simulink model "singal_three"  (R2023b)
settings: Solver=VariableStepAuto  StartTime=0.0  StopTime=1  RelTol=1e-3
InitFcn:
  | fc=20000;
  | Ts=1/20000;
libraries: spsSeriesRLCBranchLib x17, spsCurrentMeasurementLib x4, spsVoltageMeasurementLib x4, simulink x2, spsUniversalBridgeLib x2, spsDCVoltageSourceLib x1, spsDiodeLib x1, spsMosfetLib x1, spsMutualInductanceLib x1, sps_lib x1
settings Model: SimulationMode=accelerator  Creator=45276  LastModifiedBy=45276

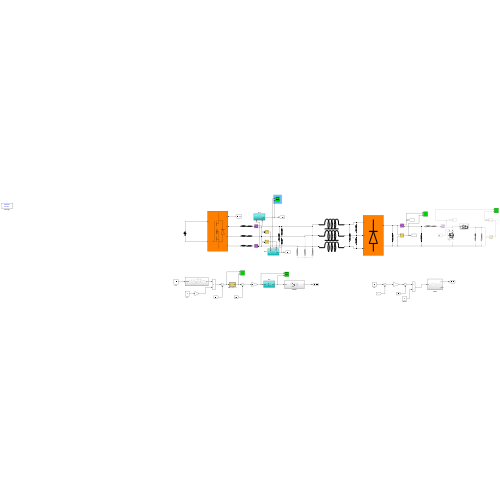
[thumbnail: Simulink's stored preview of the top-level diagram]
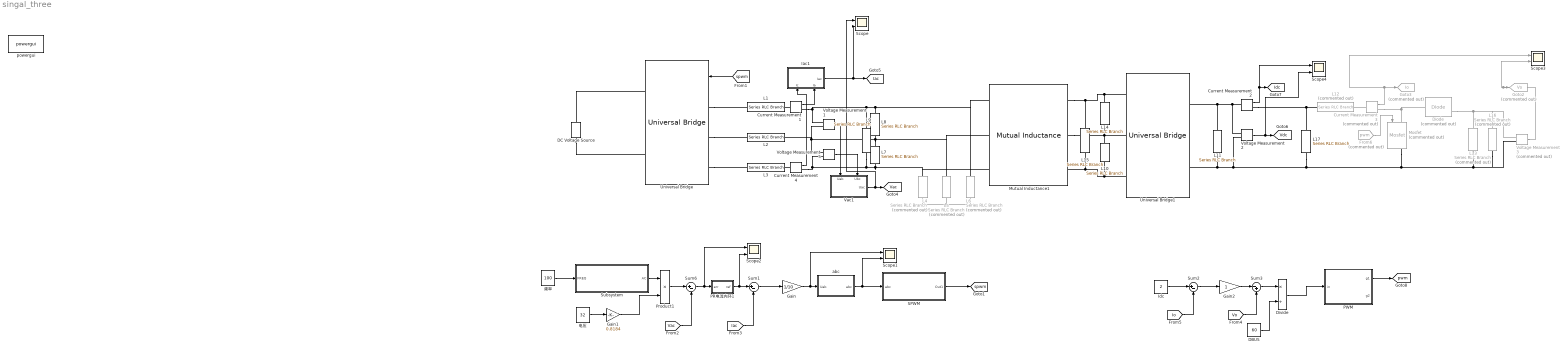
== system singal_three ==
  Current Measurement1 : spsCurrentMeasurementLib/Current Measurement  PhasorSimulation=off  OutputType=Complex  PSBequivalent=0
  Current Measurement2 : spsCurrentMeasurementLib/Current Measurement  PhasorSimulation=off  OutputType=Complex  PSBequivalent=0
  Current Measurement3 : spsCurrentMeasurementLib/Current Measurement  Commented=on  PhasorSimulation=off  OutputType=Complex  PSBequivalent=0
  Current Measurement4 : spsCurrentMeasurementLib/Current Measurement  PhasorSimulation=off  OutputType=Complex  PSBequivalent=0
  DBUS : Constant  Value=60
  DC Voltage Source : spsDCVoltageSourceLib/DC Voltage Source  Amplitude=60  Measurements=None
  Diode : spsDiodeLib/Diode  Commented=on  Ron=0.001  Lon=0  Vf=0.8  IC=0  UseSnubber=0  Rs=500  Cs=250e-9  Measurements=on
  Divide : Product  Inputs=*/
  From6 : From  Commented=on  GotoTag=pwm  TagVisibility=global
  Gain : Gain  Gain=1/10
  Gain1 : Gain  Gain=0.8184
  Gain2 : Gain
  Goto2 : Goto  Commented=on  GotoTag=Vo  TagVisibility=global
  Goto3 : Goto  Commented=on  GotoTag=Io  TagVisibility=global
  Iac1 : Subsystem
      settings: PortSchema="{\"entries\":[{\"content\":{\"sides\":[{\"content\":{\"connectorIds\":[\"In1\",\"In2\"]},\"type\":\"ConnectorPlacement.EquallySpacedRectSide\",\"uuid\":\"58c40194-9a95-4e39-952e-f878bde7484e\"},{\"content\":{\"connectorIds\":[],\"side\":\"RIGHT\"},\"type\":\"ConnectorPlacement.EquallySpacedRectSide\",\"uuid\":\"f51692e8-3ff2-4d72-808d-3667196a4526\"},{\"content\":{\"connectorIds\":[],\"side\":\"TOP\"},\"type\":\"ConnectorPlacement.EquallySpacedRectSide\",\"uuid\":\"0aab136b-5da5-45c4-8998-999ebe8b7f2f\"},{\"content\":{\"connectorIds\":[\"Out1\"],\"side\":\"BOTTOM\"},\"type\":\"ConnectorPlacement.EquallySpacedRectSide\",\"uuid\":\"32f5f4a5-4ebb-496b-828d-b973bd46b44e\"}]},\"type\":\"ConnectorPlacement.EquallySpacedConnector\",\"uuid\":\"3ef81af7-d426-47fb-88e3-e33e58eebb83\"}],\"packageUris\":[\"http://schema.mathworks.com/mf0/Connector/R2020b\"],\"version\":\"1.0\"}"
  Idc : Constant  Value=2
  L1 : spsSeriesRLCBranchLib/Series RLC Branch  LConnTagsString=__new0  RConnTagsString=__new0  BranchType=RL  Resistance=0.001  Inductance=470e-6  SetiL0=off  InitialCurrent=0  Capacitance=3e-6  Setx0=off  InitialVoltage=0  Measurements=None
  L{7..10,14..15} (6 alike) : spsSeriesRLCBranchLib/Series RLC Branch  LConnTagsString=__new0  RConnTagsString=__new0  BranchType=RC  Resistance=0.001  Inductance=2e-3  SetiL0=off  InitialCurrent=0  Capacitance=3e-6  Setx0=off  InitialVoltage=0  Measurements=None
  L11 : spsSeriesRLCBranchLib/Series RLC Branch  LConnTagsString=__new0  RConnTagsString=__new0  BranchType=RC  Resistance=0.001  Inductance=2e-3  SetiL0=off  InitialCurrent=0  Capacitance=3e-3  Setx0=off  InitialVoltage=0  Measurements=None
  L12 : spsSeriesRLCBranchLib/Series RLC Branch  Commented=on  LConnTagsString=__new0  RConnTagsString=__new0  BranchType=RL  Resistance=0.001  Inductance=470e-6  SetiL0=off  InitialCurrent=0  Capacitance=3e-6  Setx0=off  InitialVoltage=0  Measurements=None
  L13 : spsSeriesRLCBranchLib/Series RLC Branch  Commented=on  LConnTagsString=__new0  RConnTagsString=__new0  BranchType=RC  Resistance=0.001  Inductance=2e-3  SetiL0=off  InitialCurrent=0  Capacitance=470e-6  Setx0=off  InitialVoltage=0  Measurements=None
  L16 : spsSeriesRLCBranchLib/Series RLC Branch  Commented=on  LConnTagsString=__new0  RConnTagsString=__new0  BranchType=R  Resistance=20  Inductance=2e-3  SetiL0=off  InitialCurrent=0  Capacitance=470e-6  Setx0=off  InitialVoltage=0  Measurements=None
  L17 : spsSeriesRLCBranchLib/Series RLC Branch  LConnTagsString=__new0  RConnTagsString=__new0  BranchType=R  Resistance=10  Inductance=2e-3  SetiL0=off  InitialCurrent=0  Capacitance=3e-3  Setx0=off  InitialVoltage=0  Measurements=None
  L2 : spsSeriesRLCBranchLib/Series RLC Branch  LConnTagsString=__new0  RConnTagsString=__new0  BranchType=RL  Resistance=0.001  Inductance=470e-6  SetiL0=off  InitialCurrent=0  Capacitance=3e-6  Setx0=off  InitialVoltage=0  Measurements=None
  L3 : spsSeriesRLCBranchLib/Series RLC Branch  LConnTagsString=__new0  RConnTagsString=__new0  BranchType=RL  Resistance=0.001  Inductance=470e-6  SetiL0=off  InitialCurrent=0  Capacitance=3e-6  Setx0=off  InitialVoltage=0  Measurements=None
  L4 : spsSeriesRLCBranchLib/Series RLC Branch  Commented=on  LConnTagsString=__new0  RConnTagsString=__new0  BranchType=R  Resistance=10  Inductance=2e-3  SetiL0=off  InitialCurrent=0  Capacitance=3e-6  Setx0=off  InitialVoltage=0  Measurements=None
  L5 : spsSeriesRLCBranchLib/Series RLC Branch  Commented=on  LConnTagsString=__new0  RConnTagsString=__new0  BranchType=R  Resistance=10  Inductance=2e-3  SetiL0=off  InitialCurrent=0  Capacitance=3e-6  Setx0=off  InitialVoltage=0  Measurements=None
  L6 : spsSeriesRLCBranchLib/Series RLC Branch  Commented=on  LConnTagsString=__new0  RConnTagsString=__new0  BranchType=R  Resistance=10  Inductance=2e-3  SetiL0=off  InitialCurrent=0  Capacitance=3e-6  Setx0=off  InitialVoltage=0  Measurements=None
  Mosfet : spsMosfetLib/Mosfet  Commented=on  Ron=0.1  Lon=0  Rd=0.01  Vfd=0  IC=0  Rs=1e5  Cs=inf  Measurements=on
  Mutual Inductance1 : spsMutualInductanceLib/Mutual Inductance  LConnTagsString=a|b|c  RConnTagsString=A|B|C  TypeOfMutual=Two or three windings with equal mutual terms  NumberOfWindings=3  SelfImpedance1=[0.01 1e-03]  SelfImpedance2=[0.01 1e-03]  ThreeWindings=on  SelfImpedance3=[0.01 1e-03]  MutualImpedance=[0.02 0.9e-03]  InductanceMatrix="[1.0 0.9  0.9 ;  0.9 1.0  0.9;  0.9 0.9 1.0 ] * 1e-3"  ResistanceMatrix="[1.0 0.9  0.9 ;  0.9 1.0  0.9;  0.9 0.9 1.0 ]"  Measurements=None
  PR电流内环1 : Subsystem  TreatAsAtomicUnit=on  mask{Kp=0.1, Kr=40, Wc=10, Upper=40, Lower=-40}
  PWM : Subsystem
  Product1 : Product
  SPWM : Subsystem
  Scope{,1..4} (5 alike) : Scope  NumInputPorts=2
  Subsystem : Subsystem
  Sum1 : Sum  Inputs=|+-
  Sum2 : Sum  Inputs=|+-
  Sum3 : Sum  Inputs=|-+
  Sum6 : Sum  Inputs=|+-
  Universal Bridge : spsUniversalBridgeLib/Universal Bridge  Arms=3  SnubberResistance=1e5  SnubberCapacitance=inf  Device=MOSFET / Diodes  Ron=1e-3  Lon=0  ForwardVoltages="[  0  0  ]"  ForwardVoltage=0  GTOparameters=[ 10e-6 , 20e-6 ]  IGBTparameters=[ 1e-6 , 2e-6 ]  Measurements=None  Measurements_2=None  converterType=Rectifier
  Universal Bridge1 : spsUniversalBridgeLib/Universal Bridge  Arms=3  SnubberResistance=1e5  SnubberCapacitance=inf  Device=Diodes  Ron=1e-3  Lon=0  ForwardVoltages="[  0  0  ]"  ForwardVoltage=0  GTOparameters=[ 10e-6 , 20e-6 ]  IGBTparameters=[ 1e-6 , 2e-6 ]  Measurements=None  Measurements_2=None  converterType=Rectifier
  Vac1 : Subsystem
      settings: PortSchema="{\"entries\":[{\"content\":{\"sides\":[{\"content\":{\"connectorIds\":[\"In1\",\"In2\"]},\"type\":\"ConnectorPlacement.EquallySpacedRectSide\",\"uuid\":\"58c40194-9a95-4e39-952e-f878bde7484e\"},{\"content\":{\"connectorIds\":[],\"side\":\"RIGHT\"},\"type\":\"ConnectorPlacement.EquallySpacedRectSide\",\"uuid\":\"f51692e8-3ff2-4d72-808d-3667196a4526\"},{\"content\":{\"connectorIds\":[],\"side\":\"TOP\"},\"type\":\"ConnectorPlacement.EquallySpacedRectSide\",\"uuid\":\"0aab136b-5da5-45c4-8998-999ebe8b7f2f\"},{\"content\":{\"connectorIds\":[\"Out1\"],\"side\":\"BOTTOM\"},\"type\":\"ConnectorPlacement.EquallySpacedRectSide\",\"uuid\":\"185ce796-68e2-4136-8080-97dc86d2ba54\"}]},\"type\":\"ConnectorPlacement.EquallySpacedConnector\",\"uuid\":\"3ef81af7-d426-47fb-88e3-e33e58eebb83\"}],\"packageUris\":[\"http://schema.mathworks.com/mf0/Connector/R2020b\"],\"version\":\"1.0\"}"
  Voltage Measurement1 : spsVoltageMeasurementLib/Voltage Measurement  PhasorSimulation=off  OutputType=Complex  PSBequivalent=0
  Voltage Measurement2 : spsVoltageMeasurementLib/Voltage Measurement  PhasorSimulation=off  OutputType=Complex  PSBequivalent=0
  Voltage Measurement3 : spsVoltageMeasurementLib/Voltage Measurement  Commented=on  PhasorSimulation=off  OutputType=Complex  PSBequivalent=0
  Voltage Measurement5 : spsVoltageMeasurementLib/Voltage Measurement  PhasorSimulation=off  OutputType=Complex  PSBequivalent=0
  abc : Subsystem
      settings: PortSchema="{\"entries\":[{\"content\":{\"sides\":[{\"content\":{},\"type\":\"ConnectorPlacement.EquallySpacedRectSide\",\"uuid\":\"58c40194-9a95-4e39-952e-f878bde7484e\"},{\"content\":{\"side\":\"RIGHT\"},\"type\":\"ConnectorPlacement.EquallySpacedRectSide\",\"uuid\":\"f51692e8-3ff2-4d72-808d-3667196a4526\"},{\"content\":{\"connectorIds\":[\"In1\"],\"side\":\"TOP\"},\"type\":\"ConnectorPlacement.EquallySpacedRectSide\",\"uuid\":\"0aab136b-5da5-45c4-8998-999ebe8b7f2f\"},{\"content\":{\"connectorIds\":[\"Out1\"],\"side\":\"BOTTOM\"},\"type\":\"ConnectorPlacement.EquallySpacedRectSide\",\"uuid\":\"32f5f4a5-4ebb-496b-828d-b973bd46b44e\"}]},\"type\":\"ConnectorPlacement.EquallySpacedConnector\",\"uuid\":\"3ef81af7-d426-47fb-88e3-e33e58eebb83\"}],\"packageUris\":[\"http://schema.mathworks.com/mf0/Connector/R2020b\"],\"version\":\"1.0\"}"
  powergui : sps_lib/powergui  Priority=1  SimulationMode=Discrete  SampleTime=2e-7  frequency=60  Iterations=50  frequencyindice=0  Pbase=100e6  ErrMax=1e-4  UnitsV=kV  UnitsW=MW  buscounter=0  FunctionMessages=off  echomessages=off  EnableUseOfTLC=off  CurrentSourceSwitches=off  DisableSnubberDevices=off  DisableRonSwitches=off  DisableVfSwitches=off  DisplayEquations=off  AutomaticDiscreteSolvers=off  SolverType=Tustin/Backward Euler (TBE)  Interpol=off  ExternalGateDelay=off  methode=off  Ts=100  x0status=blocks  SPID=on  SwTol=0  HookPort=off  NonlinearTolerance=1e-4  nMaxIteration=100  ContinueOnMaxIteration=off  RestoreLinks=warning  ResistiveCurrentMeasurement=off  Frange=[0:2:500]  Ylog=off  Xlog=on  ShowGrid=off  save=off  variable=ZData  structure=0  ZoomFFT=off  StartTime=0.0  cycles=1  DisplayStyle=1  fundamental=60  FreqAxis=off  MaxFrequency=1000  frequencyindicesteady=1  RmsSteady=1  display=off
  电压 : Constant  Value=32
  频率 : Constant  Value=100
  tag scope: Iac=global, Idc=global, Vac=global, Vdc=global, pwm=global, spwm=global
  wires:
  [spwm] -> Universal Bridge/1
  频率/1 -> Subsystem/1(FREQ)
  Subsystem/1(AC) -> Product1/1
  PR电流内环1/1(ref) -> Scope2/2, Sum1/1
  Sum6/1 -> Scope2/1, PR电流内环1/1(err)
  Product1/1 -> Sum6/1
  电压/1 -> Gain1/1
  Vac1/1(Uac) -> Scope/1, [Vac]
  Voltage Measurement5/1 -> Vac1/2(Ubc)
  Iac1/1(Iac) -> Scope/2, [Iac]
  Voltage Measurement1/1 -> Vac1/1(Uab)
  Current Measurement1/1 -> Iac1/2(Ia)
  Current Measurement4/1 -> Iac1/1(Ic)
  [Vac] -> Sum6/2
  [Iac] -> Sum1/2
  Sum1/1 -> Gain/1
  SPWM/1(Out1) -> [spwm]
  Gain/1 -> Scope1/1, abc/1(Uab)
  abc/1(abc) -> SPWM/1(abc), Scope1/2
  Voltage Measurement3/1 -> Scope3/2, Goto2/1
  Current Measurement3/1 -> Scope3/1, Goto3/1
  Voltage Measurement2/1 -> Scope4/2, [Vdc]
  Current Measurement2/1 -> Scope4/1, [Idc]
  [Io] -> Sum2/2
  Sum2/1 -> Gain2/1
  Divide/1 -> PWM/1(in)
  PWM/1(g1) -> [pwm]
  From6/1 -> Mosfet/1
  Idc/1 -> Sum2/1
  Gain2/1 -> Sum3/1
  Sum3/1 -> Divide/1
  [Vo] -> Sum3/2
  DBUS/1 -> Divide/2
  Gain1/1 -> Product1/2
  connections:
  Universal Bridge/LConn3 -- L3/RConn1
  Universal Bridge/LConn2 -- L2/RConn1
  Universal Bridge/LConn1 -- L1/RConn1
  L7/RConn1 -- Mutual Inductance1/LConn3 -- L4/LConn1 -- L9/RConn1 -- Voltage Measurement5/LConn2 -- Current Measurement4/RConn1
  L8/LConn1 -- L6/LConn1 -- Mutual Inductance1/LConn1 -- L9/LConn1 -- Current Measurement1/RConn1 -- Voltage Measurement1/LConn1
  L7/LConn1 -- Mutual Inductance1/LConn2 -- L5/LConn1 -- L8/RConn1 -- Voltage Measurement1/LConn2 -- L2/LConn1 -- Voltage Measurement5/LConn1
  DC Voltage Source/LConn1 -- Universal Bridge/RConn2
  Current Measurement1/LConn1 -- L1/LConn1
  Current Measurement4/LConn1 -- L3/LConn1
  Voltage Measurement2/LConn1 -- Current Measurement2/LConn1 -- L11/LConn1 -- Universal Bridge1/RConn1
  Current Measurement2/RConn1 -- L17/LConn1 -- L12/RConn1
  Diode/LConn1 -- Current Measurement3/RConn1 -- Mosfet/LConn1
  DC Voltage Source/RConn1 -- Universal Bridge/RConn1
  Current Measurement3/LConn1 -- L12/LConn1
  Mutual Inductance1/RConn1 -- L15/LConn1 -- L14/LConn1 -- Universal Bridge1/LConn1
  Mutual Inductance1/RConn2 -- L14/RConn1 -- L10/LConn1 -- Universal Bridge1/LConn2
  Universal Bridge1/LConn3 -- L10/RConn1 -- L15/RConn1 -- Mutual Inductance1/RConn3
  Diode/RConn1 -- L16/LConn1 -- Voltage Measurement3/LConn1 -- L13/LConn1
  L11/RConn1 -- L17/RConn1 -- L16/RConn1 -- Voltage Measurement3/LConn2 -- L13/RConn1 -- Mosfet/RConn1 -- Voltage Measurement2/LConn2 -- Universal Bridge1/RConn2
  L4/RConn1 -- L5/RConn1 -- L6/RConn1

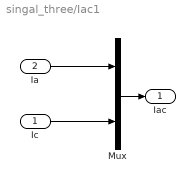
== system singal_three/Iac1 ==
  Ic : Inport
  Ia : Inport  Port=2
  Mux : Mux  Inputs=2
  Iac : Outport
  wires:
  Mux/1 -> Iac/1
  Ic/1 -> Mux/2
  Ia/1 -> Mux/1

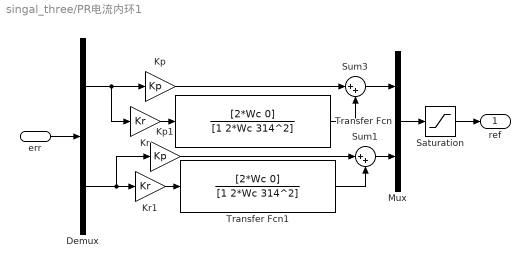
== system singal_three/PR电流内环1 ==
  err : Inport
  Demux : Demux  Outputs=2
  Kp : Gain  Gain=Kp
  Kp1 : Gain  Gain=Kp
  Kr : Gain  Gain=Kr
  Kr1 : Gain  Gain=Kr
  Mux : Mux  Inputs=2
  Saturation : Saturate  UpperLimit=Upper  LowerLimit=Lower
  Sum1 : Sum  Inputs=|++
  Sum3 : Sum  Inputs=|++
  Transfer Fcn : TransferFcn  Numerator=[2*Wc 0]  Denominator=[1 2*Wc 314^2]
  Transfer Fcn1 : TransferFcn  Numerator=[2*Wc 0]  Denominator=[1 2*Wc 314^2]
  ref : Outport
  wires:
  Mux/1 -> Saturation/1
  Sum1/1 -> Mux/2
  Kr1/1 -> Transfer Fcn1/1
  Transfer Fcn1/1 -> Sum1/2
  Kp1/1 -> Sum1/1
  Demux/2 -> Kp1/1, Kr1/1
  Sum3/1 -> Mux/1
  Demux/1 -> Kp/1, Kr/1
  err/1 -> Demux/1
  Kp/1 -> Sum3/1
  Saturation/1 -> ref/1
  Transfer Fcn/1 -> Sum3/2
  Kr/1 -> Transfer Fcn/1

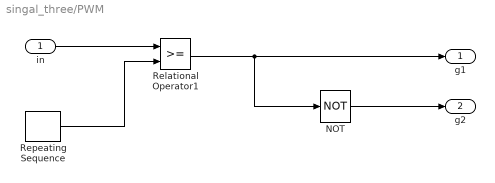
== system singal_three/PWM ==
  in : Inport
  NOT : Logic  Operator=NOT  IconShape=distinctive  AllPortsSameDT=off  OutDataTypeStr=boolean
  Relational Operator1 : RelationalOperator  OutDataTypeStr=boolean  RndMeth=Simplest  InputSameDT=off
  Repeating Sequence : simulink/Sources/Repeating Sequence  rep_seq_t=[0 20000/2 20000]  rep_seq_y=[0 1 0]
  g1 : Outport
  g2 : Outport  Port=2
  wires:
  Relational Operator1/1 -> g1/1, NOT/1
  in/1 -> Relational Operator1/1
  Repeating Sequence/1 -> Relational Operator1/2
  NOT/1 -> g2/1

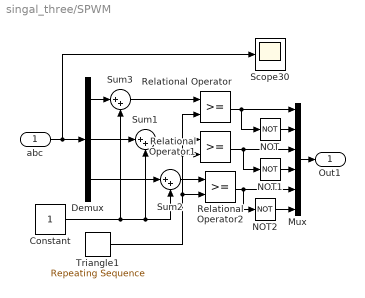
== system singal_three/SPWM ==
  abc : Inport
  Constant : Constant
  Demux : Demux  Outputs=3
  Mux : Mux  Inputs=6
  NOT : Logic  Operator=NOT  IconShape=distinctive  AllPortsSameDT=off  OutDataTypeStr=boolean
  NOT1 : Logic  Operator=NOT  IconShape=distinctive  AllPortsSameDT=off  OutDataTypeStr=boolean
  NOT2 : Logic  Operator=NOT  IconShape=distinctive  AllPortsSameDT=off  OutDataTypeStr=boolean
  Relational Operator : RelationalOperator  OutDataTypeStr=boolean  RndMeth=Simplest  InputSameDT=off
  Relational Operator1 : RelationalOperator  OutDataTypeStr=boolean  RndMeth=Simplest  InputSameDT=off
  Relational Operator2 : RelationalOperator  OutDataTypeStr=boolean  RndMeth=Simplest  InputSameDT=off
  Scope30 : Scope
  Sum1 : Sum  Inputs=|++
  Sum2 : Sum  Inputs=|++
  Sum3 : Sum  Inputs=|++
  Triangle1 : simulink/Sources/Repeating Sequence  rep_seq_t=[0 1/20000/2 1/20000]  rep_seq_y=[0 2 0]
  Out1 : Outport
  wires:
  Mux/1 -> Out1/1
  NOT2/1 -> Mux/6
  NOT1/1 -> Mux/4
  Relational Operator2/1 -> Mux/5, NOT2/1
  Relational Operator1/1 -> Mux/3, NOT1/1
  Relational Operator/1 -> Mux/1, NOT/1
  NOT/1 -> Mux/2
  Triangle1/1 -> Relational Operator/2, Relational Operator1/2, Relational Operator2/2
  abc/1 -> Scope30/1, Demux/1
  Demux/1 -> Sum3/1
  Sum3/1 -> Relational Operator/1
  Demux/2 -> Sum1/1
  Sum1/1 -> Relational Operator1/1
  Demux/3 -> Sum2/1
  Sum2/1 -> Relational Operator2/1
  Constant/1 -> Sum2/2, Sum1/2, Sum3/2

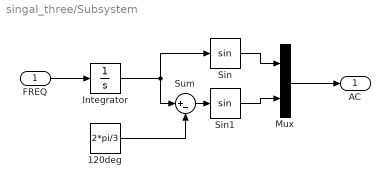
== system singal_three/Subsystem ==
  FREQ : Inport
  120deg : Constant  Value=2*pi/3
  Integrator : Integrator  WrapState=on  WrappedStateUpperValue=2*pi  WrappedStateLowerValue=0
  Mux : Mux  Inputs=2
  Sin : Trigonometry
  Sin1 : Trigonometry
  Sum : Sum  Inputs=|+-
  AC : Outport
  wires:
  FREQ/1 -> Integrator/1
  Sin/1 -> Mux/1
  Mux/1 -> AC/1
  120deg/1 -> Sum/2
  Integrator/1 -> Sin/1, Sum/1
  Sum/1 -> Sin1/1
  Sin1/1 -> Mux/2

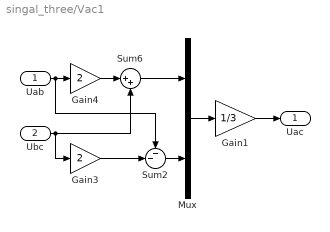
== system singal_three/Vac1 ==
  Uab : Inport
  Ubc : Inport  Port=2
  Gain1 : Gain  Gain=1/3
  Gain3 : Gain  Gain=2
  Gain4 : Gain  Gain=2
  Mux : Mux  Inputs=2
  Sum2 : Sum  Inputs=--|
  Sum6 : Sum  Inputs=|++
  Uac : Outport
  wires:
  Gain1/1 -> Uac/1
  Mux/1 -> Gain1/1
  Gain3/1 -> Sum2/2
  Sum2/1 -> Mux/2
  Ubc/1 -> Gain3/1, Sum6/2
  Gain4/1 -> Sum6/1
  Uab/1 -> Gain4/1, Sum2/1
  Sum6/1 -> Mux/1

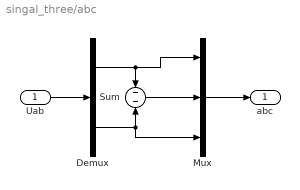
== system singal_three/abc ==
  Uab : Inport
  Demux : Demux  Outputs=2
  Mux : Mux  Inputs=3
  Sum : Sum  Inputs=-|-
  abc : Outport
  wires:
  Uab/1 -> Demux/1
  Demux/1 -> Mux/1, Sum/1
  Demux/2 -> Mux/3, Sum/2
  Sum/1 -> Mux/2
  Mux/1 -> abc/1
